simulink model "test_adc"  (R2016a)
settings: Solver=FixedStepDiscrete  StartTime=0.0  StopTime=inf  RelTol=1e-3
libraries: c280xlib x2, c2802xlib x1, c2837xDlib x1
settings Model: SimulationMode=external  ExtModeTrigDuration=8  Creator=ric  LastModifiedBy=ric
settings OptimizationCC: OptimizeModelRefInitCode=on  LifeSpan=1  MaxStackSize=512
settings HardwareCC: ProdBitPerChar=16  ProdBitPerInt=16  ProdBitPerPointer=32  ProdLargestAtomicInteger=Integer  ProdLargestAtomicFloat=None  ProdWordSize=16  ProdLongLongMode=on  ProdHWDeviceType=Texas Instruments->C2000
settings RTWCC: SystemTargetFile=ert.tlc  HardwareBoard=TI Delfino F2837xS  TemplateMakefile=ert_default_tmf  GenerateReport=on  RTWVerbose=off  Toolchain=Texas Instruments Code Composer Studio v6 (C2000)  IncludeHyperlinkInReport=on  LaunchReport=on  GenerateTraceInfo=on  GenerateTraceReport=on  GenerateTraceReportSl=on  GenerateTraceReportSf=on  GenerateTraceReportEml=on
settings CodeAppCC: ForceParamTrailComments=on  IgnoreCustomStorageClasses=off  OperatorAnnotations=on  SimulinkDataObjDesc=on  SFDataObjDesc=on  MATLABFcnDesc=on  InsertBlockDesc=on  MATLABSourceComments=on
settings ERTTargetCC: CodeReplacementLibrary=TI C28x

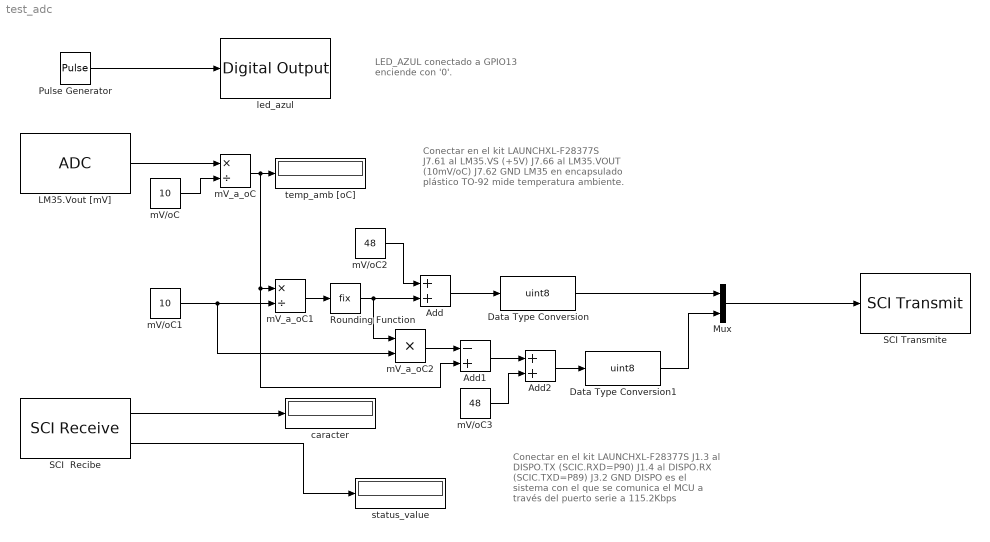
== system test_adc ==
  note: LED_AZUL conectado a GPIO13
      | enciende con '0'.
  note: Conectar en el kit LAUNCHXL-F28377S
      | J1.3 al DISPO.TX (SCIC.RXD=P90)
      | J1.4 al DISPO.RX (SCIC.TXD=P89)
      | J3.2 GND
      | DISPO es el sistema con el que se
      | comunica el MCU a través del puerto
      | serie a 115.2Kbps
  note: Conectar en el kit LAUNCHXL-F28377S
      | J7.61 al LM35.VS (+5V)
      | J7.66 al LM35.VOUT (10mV/oC)
      | J7.62 GND
      | LM35 en encapsulado plástico TO-92
      | mide temperatura ambiente.
  Add : Sum
  Add1 : Sum  Inputs=-+
  Add2 : Sum
  Data Type Conversion : DataTypeConversion  OutDataTypeStr=uint8
  Data Type Conversion1 : DataTypeConversion  OutDataTypeStr=uint8
  LM35.Vout [mV] : c2802xlib/ADC  ADCModule=B  samplingMode=Single sample mode  ADCResolution=12-bit (Single-ended input)  useSOC1=SOC0  useSOC2=SOC0_SOC1  SOCAcquisitionWindow=7  SOCTriggerSource=Software  SOCInterruptTrigger=No ADCINT  Ts=0.001  dType=uint16  postInterrupt=off  interruptSel=ADCINT1  ADCINTContinuous=on  endma=off  chdma=1  blkParamProc=C2000_Type4  conv1=ADCINA0  conv2=ADCINA0 and ADCINB0  conv1_Type4=ADCIN5  conv2_Type4=ADCIN0 and ADCIN1
  Mux : Mux  Inputs=2
  Pulse Generator : DiscretePulseGenerator  PulseType=Time based  Period=1  PulseWidth=50
  Rounding Function : Rounding  Operator=fix
  SCI  Recibe : c280xlib/SCI Receive  sciModule=C  dataHead=''  dataTail=''  dataType=uint8  dataDim=1  initValue=0  errOption=Output custom value  errValue=0  sampleTime=0.01  outputStatus=on  postInterrupt=off  numFifo=1
  SCI Transmite : c280xlib/SCI Transmit  sciModule=C  dataHead=''  dataTail='\r\n'  postInterrupt=off  numFifo=1
  caracter : Display
  led_azul : c2837xDlib/Digital Output  GPIO_Number=GPIO8~GPIO15  GPIO_Bit0=off  GPIO_BIT0_Toggle=off  GPIO_Bit1=off  GPIO_BIT1_Toggle=off  GPIO_Bit2=off  GPIO_BIT2_Toggle=off  GPIO_Bit3=off  GPIO_BIT3_Toggle=off  GPIO_Bit4=off  GPIO_BIT4_Toggle=off  GPIO_Bit5=on  GPIO_BIT5_Toggle=off  GPIO_Bit6=off  GPIO_BIT6_Toggle=off  GPIO_Bit7=off  GPIO_BIT7_Toggle=off
  mV/oC : Constant  Value=10
  mV/oC1 : Constant  Value=10
  mV/oC2 : Constant  Value=48
  mV/oC3 : Constant  Value=48
  mV_a_oC : Product  Inputs=*/
  mV_a_oC1 : Product  Inputs=*/
  mV_a_oC2 : Product  Inputs=**
  status_value : Display
  temp_amb [oC] : Display
  wires:
  Pulse Generator/1 -> led_azul/1
  SCI  Recibe/2 -> status_value/1
  mV_a_oC/1 -> Add1/2, mV_a_oC1/1, temp_amb [oC]/1
  LM35.Vout [mV]/1 -> mV_a_oC/1
  mV/oC/1 -> mV_a_oC/2
  mV/oC1/1 -> mV_a_oC2/2, mV_a_oC1/2
  mV/oC2/1 -> Add/1
  SCI  Recibe/1 -> caracter/1
  Add/1 -> Data Type Conversion/1
  mV_a_oC2/1 -> Add1/1
  Add1/1 -> Add2/1
  mV/oC3/1 -> Add2/2
  Add2/1 -> Data Type Conversion1/1
  Mux/1 -> SCI Transmite/1
  Data Type Conversion/1 -> Mux/1
  Data Type Conversion1/1 -> Mux/2
  mV_a_oC1/1 -> Rounding Function/1
  Rounding Function/1 -> mV_a_oC2/1, Add/2
